simulink model "CP_ContrSys_Lin_a_n9945008"  (R2018b)
settings: Solver=VariableStepAuto  StartTime=0.0  StopTime=5  RelTol=1e-3
values from neighbouring files (symbols this model uses):
  Aa = [ 0 ,       0            , 1 , 0 ... (first row only)    [CP_ContrSys_Lin_a_MainFile_n9945008.m]
  Ba = [0;0;1/Mc;-1/(l*Mc)]    [CP_ContrSys_Lin_a_MainFile_n9945008.m]
  Ca = [1,0,0,0 ... (first row only)    [CP_ContrSys_Lin_a_MainFile_n9945008.m]
  Ka = place(Aa,Ba, [-3,-4,-5,-6])    [CP_ContrSys_Lin_a_MainFile_n9945008.m]
  La = place(Aa',Ca', [-63,-64,-65,-66])'    [CP_ContrSys_Lin_a_MainFile_n9945008.m]
  x0 = [0.2 -50*pi/180 0 0]'    [CP_ContrSys_Lin_a_MainFile_n9945008.m]
settings Model: Creator=n9945008  LastModifiedBy=n9945008

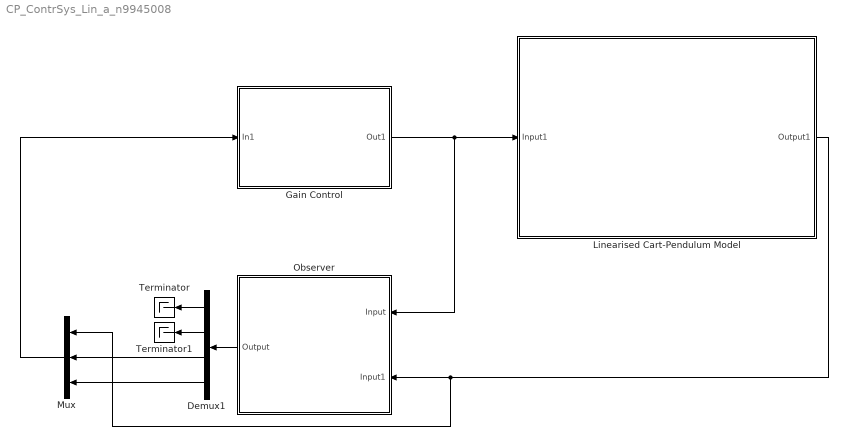
== system CP_ContrSys_Lin_a_n9945008 ==
  Demux1 : Demux
  Gain Control : Subsystem
  "Linearised Cart-Pendulum Model " : Subsystem
  Mux : Mux  Inputs=3
  Observer : Subsystem
  Terminator : Terminator
  Terminator1 : Terminator
  wires:
  Gain Control/1(Out1) -> "Linearised Cart-Pendulum Model "/1(Input1), Observer/1(Input)
  Observer/1(Output) -> Demux1/1
  Demux1/1 -> Terminator/1
  Demux1/2 -> Terminator1/1
  Demux1/3 -> Mux/2
  Demux1/4 -> Mux/3
  Mux/1 -> Gain Control/1(In1)
  "Linearised Cart-Pendulum Model "/1(Output1) -> Mux/1, Observer/2(Input1)

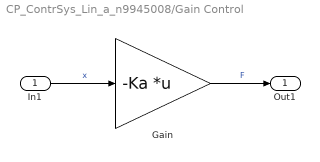
== system CP_ContrSys_Lin_a_n9945008/Gain Control ==
  In1 : Inport
  Gain : Gain  Gain=-Ka  Multiplication=Matrix(K*u)
  Out1 : Outport
  wires:
  In1/1 -> Gain/1  "x"
  Gain/1 -> Out1/1  "F"

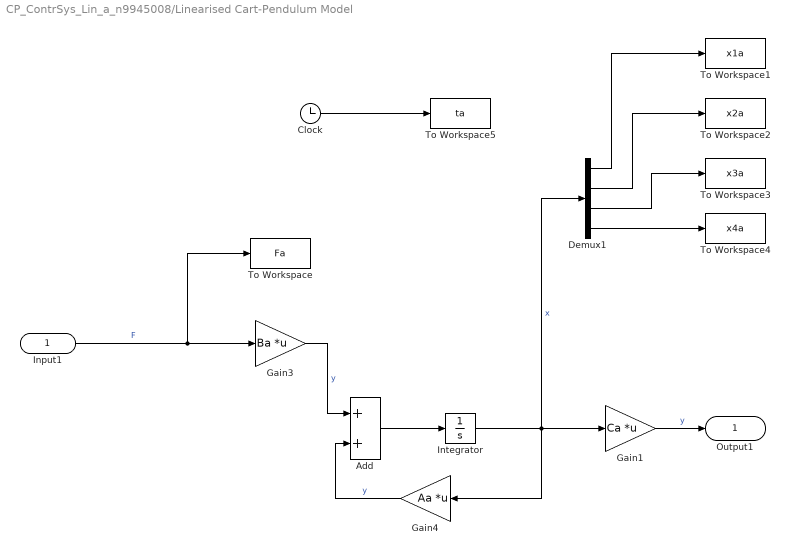
== system CP_ContrSys_Lin_a_n9945008/Linearised Cart-Pendulum Model  ==
  Input1 : Inport
  Add : Sum  Inputs=2
  Clock : Clock
  Demux1 : Demux
  Gain1 : Gain  Gain=Ca  Multiplication=Matrix(K*u)
  Gain3 : Gain  Gain=Ba  Multiplication=Matrix(K*u)
  Gain4 : Gain  Gain=Aa  Multiplication=Matrix(K*u)
  Integrator : Integrator  InitialCondition=x0
  To Workspace : ToWorkspace  VariableName=Fa  SampleTime=-1
      settings: Save2DSignal=2-D array (concatenate along first dimension)
  To Workspace1 : ToWorkspace  VariableName=x1a  SampleTime=-1
      settings: Save2DSignal=2-D array (concatenate along first dimension)
  To Workspace2 : ToWorkspace  VariableName=x2a  SampleTime=-1
      settings: Save2DSignal=2-D array (concatenate along first dimension)
  To Workspace3 : ToWorkspace  VariableName=x3a  SampleTime=-1
      settings: Save2DSignal=2-D array (concatenate along first dimension)
  To Workspace4 : ToWorkspace  VariableName=x4a  SampleTime=-1
      settings: Save2DSignal=2-D array (concatenate along first dimension)
  To Workspace5 : ToWorkspace  VariableName=ta  SampleTime=-1
      settings: Save2DSignal=2-D array (concatenate along first dimension)
  Output1 : Outport
  wires:
  Gain1/1 -> Output1/1  "y"
  Add/1 -> Integrator/1
  Demux1/3 -> To Workspace3/1
  Integrator/1 -> Gain4/1, Gain1/1, Demux1/1  "x"
  Demux1/2 -> To Workspace2/1
  Clock/1 -> To Workspace5/1
  Gain3/1 -> Add/1  "y"
  Gain4/1 -> Add/2  "y"
  Demux1/4 -> To Workspace4/1
  Input1/1 -> To Workspace/1, Gain3/1  "F"
  Demux1/1 -> To Workspace1/1

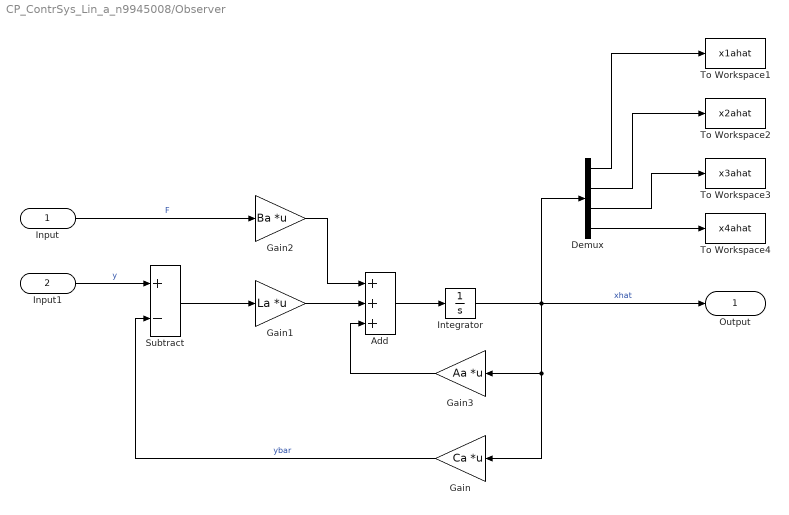
== system CP_ContrSys_Lin_a_n9945008/Observer ==
  Input : Inport
  Input1 : Inport  Port=2
  Add : Sum  Inputs=+++
  Demux : Demux
  Gain : Gain  Gain=Ca  Multiplication=Matrix(K*u)
  Gain1 : Gain  Gain=La  Multiplication=Matrix(K*u)
  Gain2 : Gain  Gain=Ba  Multiplication=Matrix(K*u)
  Gain3 : Gain  Gain=Aa  Multiplication=Matrix(K*u)
  Integrator : Integrator  InitialCondition=x0
  Subtract : Sum  Inputs=+-
  To Workspace1 : ToWorkspace  VariableName=x1ahat  SampleTime=-1
      settings: Save2DSignal=2-D array (concatenate along first dimension)
  To Workspace2 : ToWorkspace  VariableName=x2ahat  SampleTime=-1
      settings: Save2DSignal=2-D array (concatenate along first dimension)
  To Workspace3 : ToWorkspace  VariableName=x3ahat  SampleTime=-1
      settings: Save2DSignal=2-D array (concatenate along first dimension)
  To Workspace4 : ToWorkspace  VariableName=x4ahat  SampleTime=-1
      settings: Save2DSignal=2-D array (concatenate along first dimension)
  Output : Outport
  wires:
  Demux/1 -> To Workspace1/1
  Demux/4 -> To Workspace4/1
  Demux/2 -> To Workspace2/1
  Demux/3 -> To Workspace3/1
  Gain/1 -> Subtract/2  "ybar"
  Input1/1 -> Subtract/1  "y"
  Subtract/1 -> Gain1/1
  Gain1/1 -> Add/2
  Input/1 -> Gain2/1  "F"
  Gain2/1 -> Add/1
  Add/1 -> Integrator/1
  Gain3/1 -> Add/3
  Integrator/1 -> Demux/1, Gain/1, Gain3/1, Output/1  "xhat"
